simulink model "viusalization"  (R2024b)
settings: Solver=ode4  StartTime=0.0  StopTime=round(time_arr(end)*100)/100  FixedStep=1e-2  RelTol=1e-3
values from neighbouring files (symbols this model uses):
  distance_arr = path.s_arr(1:N+1)    [backwards_euler.m]    (also in circular_tube_complete_3d_model.m; complete_3d_model.m; full_3d_model.m; model_in_wind_frame.m)
  ephi_arr = sol.value(ephi)    [backwards_euler.m]    (also in circular_tube_complete_3d_model.m; complete_3d_model.m; full_3d_model.m; model_in_wind_frame.m)
  epsi_arr = sol.value(epsi)    [backwards_euler.m]    (also in circular_tube_complete_3d_model.m; complete_3d_model.m; full_3d_model.m; model_in_wind_frame.m)
  ethe_arr = sol.value(ethe)    [backwards_euler.m]    (also in circular_tube_complete_3d_model.m; complete_3d_model.m; full_3d_model.m; model_in_wind_frame.m)
  path = load('alternative_ellipse_ptf')    [backwards_euler.m]    (also in circular_tube_complete_3d_model.m = load('ellipse_2d.mat'); complete_3d_model.m = load('circle_2d.mat'); full_3d_model.m = load('three_d_infinity.mat'); model_in_wind_frame.m = load('circle_2d.mat'))
  time_arr = sol.value(t)    [backwards_euler.m]    (also in circular_tube_complete_3d_model.m; complete_3d_model.m; full_3d_model.m; model_in_wind_frame.m)
  x_arr = x    [alternative_ptf_ellipse.m]    (also in alternative_ptf_generic.m; alternative_ptf_trefoil.m; arc_2d_creation.m = [x_arr, p(1)]; backwards_euler.m = zeros(1,length(distance_arr)))
  y_arr = y    [alternative_ptf_ellipse.m]    (also in alternative_ptf_generic.m; alternative_ptf_trefoil.m; arc_2d_creation.m = [y_arr, p(2)]; backwards_euler.m = zeros(1,length(distance_arr)))
  z_arr = z    [alternative_ptf_ellipse.m]    (also in alternative_ptf_generic.m; alternative_ptf_trefoil.m; arc_2d_creation.m = [z_arr, p(3)]; backwards_euler.m = zeros(1,length(distance_arr)))
libraries: aerolibutil x2, vrlib x1
settings Model: PacingRate=0.010000  Creator=bugrauckol  LastModifiedBy=bugrauckol

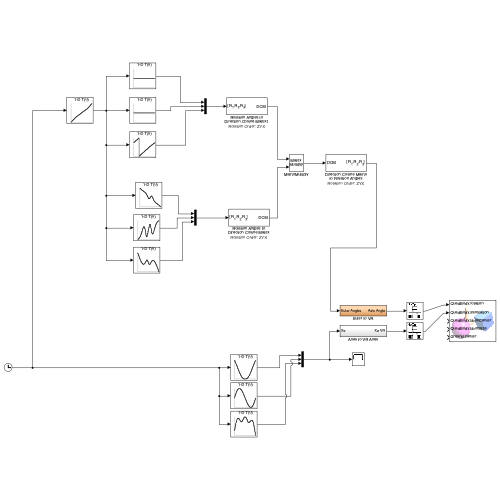
[thumbnail: Simulink's stored preview of the top-level diagram]
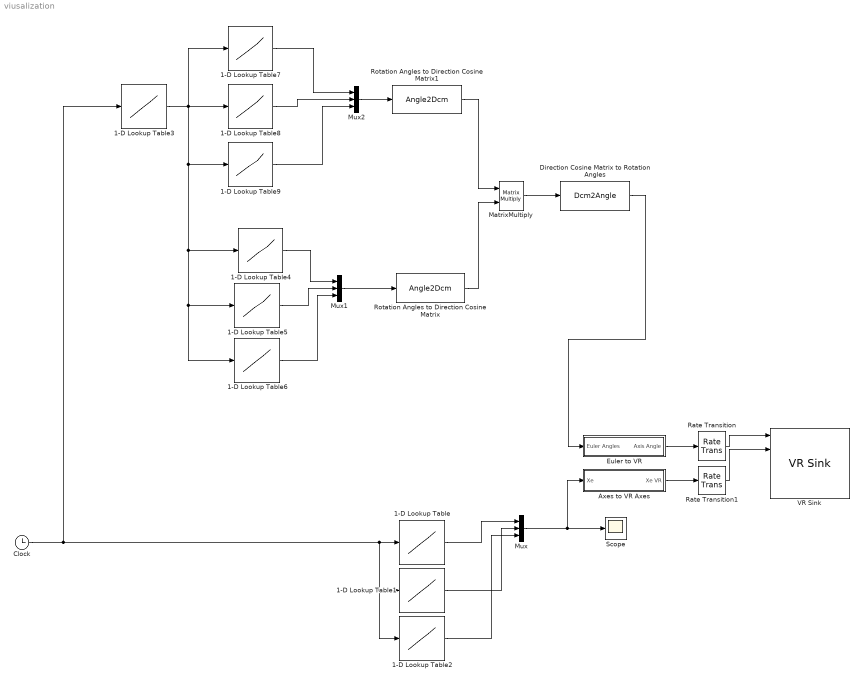
== system viusalization ==
  1-D Lookup Table : Lookup_n-D  NumberOfTableDimensions=1  BreakpointsForDimension1=time_arr  Table=x_arr  InternalRulePriority=Speed  RndMeth=Simplest
  1-D Lookup Table1 : Lookup_n-D  NumberOfTableDimensions=1  BreakpointsForDimension1=time_arr  Table=y_arr  InternalRulePriority=Speed  RndMeth=Simplest
  1-D Lookup Table2 : Lookup_n-D  NumberOfTableDimensions=1  BreakpointsForDimension1=time_arr  Table=z_arr  InternalRulePriority=Speed  RndMeth=Simplest
  1-D Lookup Table3 : Lookup_n-D  NumberOfTableDimensions=1  BreakpointsForDimension1=time_arr  Table=distance_arr  InternalRulePriority=Speed  RndMeth=Simplest
  1-D Lookup Table4 : Lookup_n-D  NumberOfTableDimensions=1  BreakpointsForDimension1=distance_arr  Table=ephi_arr  InternalRulePriority=Speed  RndMeth=Simplest
  1-D Lookup Table5 : Lookup_n-D  NumberOfTableDimensions=1  BreakpointsForDimension1=distance_arr  Table=ethe_arr  InternalRulePriority=Speed  RndMeth=Simplest
  1-D Lookup Table6 : Lookup_n-D  NumberOfTableDimensions=1  BreakpointsForDimension1=distance_arr  Table=epsi_arr  InternalRulePriority=Speed  RndMeth=Simplest
  1-D Lookup Table7 : Lookup_n-D  NumberOfTableDimensions=1  BreakpointsForDimension1=distance_arr  Table=path.roll_arr  InternalRulePriority=Speed  RndMeth=Simplest
  1-D Lookup Table8 : Lookup_n-D  NumberOfTableDimensions=1  BreakpointsForDimension1=distance_arr  Table=path.pitch_arr  InternalRulePriority=Speed  RndMeth=Simplest
  1-D Lookup Table9 : Lookup_n-D  NumberOfTableDimensions=1  BreakpointsForDimension1=distance_arr  Table=path.yaw_arr  InternalRulePriority=Speed  RndMeth=Simplest
  Axes to VR Axes : Subsystem
  Clock : Clock
  Direction Cosine Matrix to Rotation Angles : Dcm2Angle
      settings: AttributesFormatString=Rotation Order: %<rotationOrder>
  Euler to VR : Subsystem
  MatrixMultiply : Product  Multiplication=Matrix(*)
  Mux : Mux  Inputs=3
  Mux1 : Mux  Inputs=3
  Mux2 : Mux  Inputs=3
  Rate Transition : RateTransition
  Rate Transition1 : RateTransition
  Rotation Angles to Direction Cosine Matrix : Angle2Dcm
      settings: AttributesFormatString=Rotation Order: %<rotationOrder>
  Rotation Angles to Direction Cosine Matrix1 : Angle2Dcm
      settings: AttributesFormatString=Rotation Order: %<rotationOrder>
  Scope : Scope
  VR Sink : vrlib/VR Sink  InstantiateOnLoad=on  SampleTime=1e-2  ViewEnable=on  RemoteChange=off  RemoteView=off  FieldsWritten=QuadBody.rotation.4.1.1.double#QuadBody.translation.3.1.1.double#QuadBody.bboxCenter.3.1.1.double#QuadBody.bboxSize.3.1.1.double#Ground.center.3.1.1.double  WorldFileName=asbFlightSimulationWorld.wrl  AutoView=off  VideoDimensions=[]  AllowVariableSize=off  FigureProperties="{'Position', 'Name', 'Viewpoint', 'CameraBound', 'CameraDirection', 'CameraPosition', 'CameraUpVector', 'ZoomFactor', 'Antialiasing', 'Headlight', 'Lighting', 'Sound', 'StatusBar', 'Stereo3D', 'Stereo3DCameraOffset', 'Stereo3DHIT', 'ToolBar', 'Textures', 'Transparency', 'Triad', 'Wireframe', 'NavZones', 'NavMode', 'NavSpeed', 'CaptureFileFormat', 'CaptureFileName', 'Record2DCompressMethod', 'Record2DCompressQuality', 'Record2D', 'Record2DFileName', 'Record2DFPS', 'NavPanel'; [1.0000000000000000e+00   1.8300000000000000e+02   7.4500000000000000e+02   7.4800000000000000e+02], '', 'Top-down view', 'on', [7.7672039864459891e-02  -1.6049274967784294e-01  -9.8397618442934465e-01], [-1.5718662623979076e+00  -5.3905003717543098e-01  -4.8880535710510840e+00], [1.2929425233409542e-01   9.8024460600577279e-01  -1.4967801678921278e-01], [2.3939204936916333e-01], 'on', 'on', 'on', 'on', 'on', 'off', [1.0000000149011612e-01], [0.0000000000000000e+00], 'on', 'on', 'on', 'none', 'off', 'off', 'fly', 'normal', 'tif', '%f_anim_%n.tif', 'auto', [7.5000000000000000e+01], 'off', '%f_anim_%n.avi', 'auto', 'halfbar'}"
  wires:
  Euler to VR/1(Axis Angle) -> Rate Transition/1
  Axes to VR Axes/1(Xe VR) -> Rate Transition1/1
  Clock/1 -> 1-D Lookup Table3/1, 1-D Lookup Table1/1, 1-D Lookup Table2/1, 1-D Lookup Table/1
  1-D Lookup Table/1 -> Mux/1
  1-D Lookup Table1/1 -> Mux/2
  1-D Lookup Table2/1 -> Mux/3
  Mux/1 -> Axes to VR Axes/1(Xe), Scope/1
  1-D Lookup Table4/1 -> Mux1/1
  1-D Lookup Table5/1 -> Mux1/2
  1-D Lookup Table6/1 -> Mux1/3
  Mux1/1 -> Rotation Angles to Direction Cosine Matrix/1
  1-D Lookup Table3/1 -> 1-D Lookup Table7/1, 1-D Lookup Table8/1, 1-D Lookup Table6/1, 1-D Lookup Table5/1, 1-D Lookup Table4/1, 1-D Lookup Table9/1
  1-D Lookup Table8/1 -> Mux2/2
  1-D Lookup Table7/1 -> Mux2/1
  1-D Lookup Table9/1 -> Mux2/3
  Rotation Angles to Direction Cosine Matrix/1 -> MatrixMultiply/2
  Rotation Angles to Direction Cosine Matrix1/1 -> MatrixMultiply/1
  Mux2/1 -> Rotation Angles to Direction Cosine Matrix1/1
  MatrixMultiply/1 -> Direction Cosine Matrix to Rotation Angles/1
  Direction Cosine Matrix to Rotation Angles/1 -> Euler to VR/1(Euler Angles)
  Rate Transition/1 -> VR Sink/1
  Rate Transition1/1 -> VR Sink/2

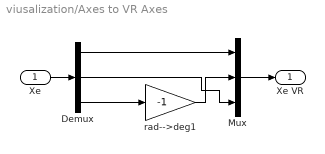
== system viusalization/Axes to VR Axes ==
  Xe : Inport
  Demux : Demux  Outputs=3
      settings: DisplayOption=none
  Mux : Mux  Inputs=3
  rad-->deg1 : Gain  Gain=-1  SaturateOnIntegerOverflow=on  OutDataTypeStr=Inherit: Same as input  ParamDataTypeStr=Inherit: Same as input
  Xe VR : Outport  VectorParamsAs1DForOutWhenUnconnected=off
  wires:
  Xe/1 -> Demux/1
  Demux/1 -> Mux/1
  Demux/3 -> rad-->deg1/1
  Mux/1 -> Xe VR/1
  rad-->deg1/1 -> Mux/2
  Demux/2 -> Mux/3

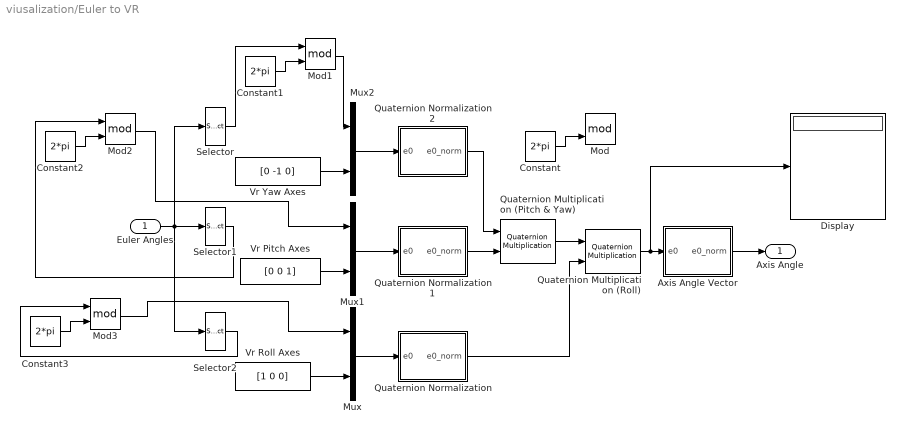
== system viusalization/Euler to VR ==
  Euler Angles : Inport
  Axis Angle Vector : Subsystem
  Constant{,1..3} (4 alike) : Constant  Value=2*pi
  Display : Display
  Mod{,1..3} (4 alike) : Math  Operator=mod
  Mux : Mux  Inputs=2
  Mux1 : Mux  Inputs=2
  Mux2 : Mux  Inputs=2
  Quaternion Multiplication (Pitch & Yaw) : aerolibutil/Quaternion Multiplication
  Quaternion Multiplication (Roll) : aerolibutil/Quaternion Multiplication
  Quaternion Normalization : Subsystem
  Quaternion Normalization1 : Subsystem
  Quaternion Normalization2 : Subsystem
  Selector : Selector  InputPortWidth=3  IndexOptions=Index vector (dialog)  Indices=[3]  OutputSizes=1
  Selector1 : Selector  InputPortWidth=3  IndexOptions=Index vector (dialog)  Indices=[2]  OutputSizes=1
  Selector2 : Selector  InputPortWidth=3  IndexOptions=Index vector (dialog)  Indices=[1]  OutputSizes=1
  Vr Pitch Axes : Constant  Value=[0 0 1]
  Vr Roll Axes : Constant  Value=[1 0 0]
  Vr Yaw Axes : Constant  Value=[0 -1 0]
  Axis Angle : Outport  VectorParamsAs1DForOutWhenUnconnected=off
  wires:
  Quaternion Multiplication (Roll)/1 -> Display/1, Axis Angle Vector/1(e0)
  Axis Angle Vector/1(e0_norm) -> Axis Angle/1
  Quaternion Normalization/1(e0_norm) -> Quaternion Multiplication (Roll)/2
  Quaternion Normalization2/1(e0_norm) -> Quaternion Multiplication (Pitch & Yaw)/1
  Quaternion Normalization1/1(e0_norm) -> Quaternion Multiplication (Pitch & Yaw)/2
  Mux2/1 -> Quaternion Normalization2/1(e0)
  Mux1/1 -> Quaternion Normalization1/1(e0)
  Mux/1 -> Quaternion Normalization/1(e0)
  Selector/1 -> Mod1/1
  Vr Yaw Axes/1 -> Mux2/2
  Vr Pitch Axes/1 -> Mux1/2
  Vr Roll Axes/1 -> Mux/2
  Euler Angles/1 -> Selector2/1, Selector1/1, Selector/1
  Quaternion Multiplication (Pitch & Yaw)/1 -> Quaternion Multiplication (Roll)/1
  Constant/1 -> Mod/2
  Constant1/1 -> Mod1/2
  Mod1/1 -> Mux2/1
  Constant2/1 -> Mod2/2
  Selector1/1 -> Mod2/1
  Mod2/1 -> Mux1/1
  Constant3/1 -> Mod3/2
  Selector2/1 -> Mod3/1
  Mod3/1 -> Mux/1

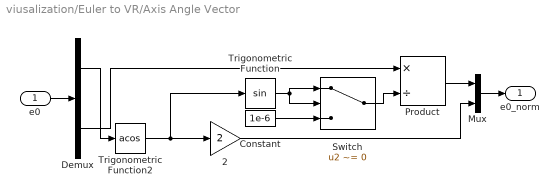
== system viusalization/Euler to VR/Axis Angle Vector ==
  e0 : Inport
  2 : Gain  Gain=2  SaturateOnIntegerOverflow=on  OutDataTypeStr=Inherit: Same as input  ParamDataTypeStr=Inherit: Same as input
  Constant : Constant  Value=1e-6
  Demux : Demux  Outputs=[1 3 ]
      settings: DisplayOption=none
  Mux : Mux  Inputs=2
  Product : Product  Inputs=*/  InputSameDT=on  SaturateOnIntegerOverflow=on  OutDataTypeStr=Inherit: Same as first input
  Switch : Switch  Criteria=u2 ~= 0  SaturateOnIntegerOverflow=off  InputSameDT=off
  Trigonometric Function : Trigonometry
  Trigonometric Function2 : Trigonometry  Operator=acos
  e0_norm : Outport  VectorParamsAs1DForOutWhenUnconnected=off
  wires:
  Demux/1 -> Trigonometric Function2/1
  Demux/2 -> Product/1
  Mux/1 -> e0_norm/1
  Product/1 -> Mux/1
  2/1 -> Mux/2
  Trigonometric Function/1 -> Switch/1, Switch/2
  Trigonometric Function2/1 -> Trigonometric Function/1, 2/1
  e0/1 -> Demux/1
  Constant/1 -> Switch/3
  Switch/1 -> Product/2

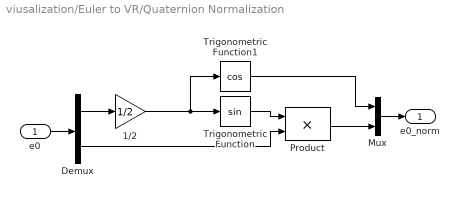
== system viusalization/Euler to VR/Quaternion Normalization ==
  e0 : Inport
  1/2 : Gain  Gain=1/2  SaturateOnIntegerOverflow=on  OutDataTypeStr=Inherit: Same as input  ParamDataTypeStr=Inherit: Same as input
  Demux : Demux  Outputs=[1 3]
      settings: DisplayOption=none
  Mux : Mux  Inputs=2
  Product : Product  InputSameDT=on  SaturateOnIntegerOverflow=on  OutDataTypeStr=Inherit: Same as first input
  Trigonometric Function : Trigonometry
  Trigonometric Function1 : Trigonometry  Operator=cos
  e0_norm : Outport  VectorParamsAs1DForOutWhenUnconnected=off
  wires:
  Trigonometric Function1/1 -> Mux/1
  Demux/2 -> Product/2
  Demux/1 -> 1/2/1
  Mux/1 -> e0_norm/1
  Product/1 -> Mux/2
  Trigonometric Function/1 -> Product/1
  1/2/1 -> Trigonometric Function1/1, Trigonometric Function/1
  e0/1 -> Demux/1

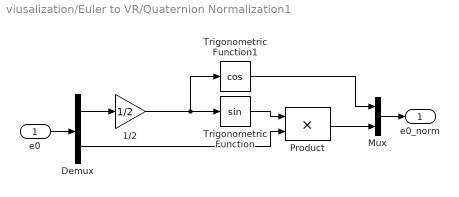
== system viusalization/Euler to VR/Quaternion Normalization1 ==
  e0 : Inport
  1/2 : Gain  Gain=1/2  SaturateOnIntegerOverflow=on  OutDataTypeStr=Inherit: Same as input  ParamDataTypeStr=Inherit: Same as input
  Demux : Demux  Outputs=[1 3]
      settings: DisplayOption=none
  Mux : Mux  Inputs=2
  Product : Product  InputSameDT=on  SaturateOnIntegerOverflow=on  OutDataTypeStr=Inherit: Same as first input
  Trigonometric Function : Trigonometry
  Trigonometric Function1 : Trigonometry  Operator=cos
  e0_norm : Outport  VectorParamsAs1DForOutWhenUnconnected=off
  wires:
  e0/1 -> Demux/1
  1/2/1 -> Trigonometric Function/1, Trigonometric Function1/1
  Trigonometric Function/1 -> Product/1
  Product/1 -> Mux/2
  Mux/1 -> e0_norm/1
  Demux/1 -> 1/2/1
  Demux/2 -> Product/2
  Trigonometric Function1/1 -> Mux/1

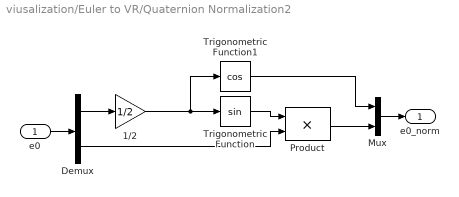
== system viusalization/Euler to VR/Quaternion Normalization2 ==
  e0 : Inport
  1/2 : Gain  Gain=1/2  SaturateOnIntegerOverflow=on  OutDataTypeStr=Inherit: Same as input  ParamDataTypeStr=Inherit: Same as input
  Demux : Demux  Outputs=[1 3]
      settings: DisplayOption=none
  Mux : Mux  Inputs=2
  Product : Product  InputSameDT=on  SaturateOnIntegerOverflow=on  OutDataTypeStr=Inherit: Same as first input
  Trigonometric Function : Trigonometry
  Trigonometric Function1 : Trigonometry  Operator=cos
  e0_norm : Outport  VectorParamsAs1DForOutWhenUnconnected=off
  wires:
  Trigonometric Function1/1 -> Mux/1
  Demux/2 -> Product/2
  Demux/1 -> 1/2/1
  Mux/1 -> e0_norm/1
  Product/1 -> Mux/2
  Trigonometric Function/1 -> Product/1
  1/2/1 -> Trigonometric Function1/1, Trigonometric Function/1
  e0/1 -> Demux/1
